simulink library "dlbsBlockTanh"  (R2025b)
settings: Solver=VariableStepAuto  StartTime=0.0  StopTime=10.0  RelTol=1e-3
libraries: dlbsBlockExtractGradientGF x1, dlbsBlockInsertGradientGF x1
settings Model: Creator=lt6037  LastModifiedBy=lt6037

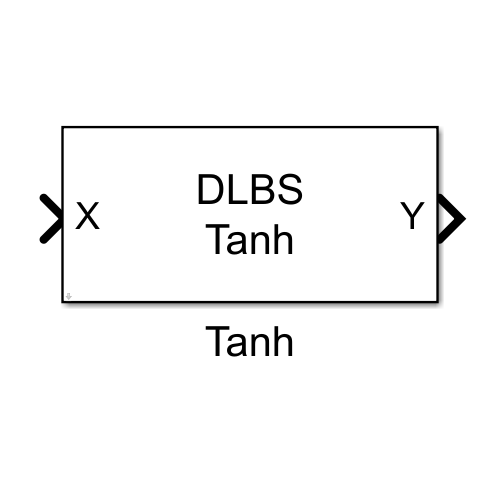
[thumbnail: Simulink's stored preview of the top-level diagram]
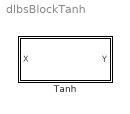
== system dlbsBlockTanh ==
  Tanh : Subsystem
      mask help: Applies the hyperbolic tangent activation to the input tensor. The operation is applied element-wise across all tensor elements.
      mask Help: web("dlbsHelpBlockTanh.html")
      mask Display: fprintf("DLBS\nTanh")

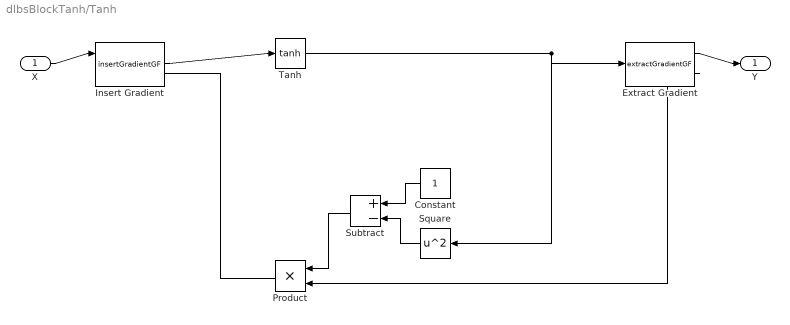
== system dlbsBlockTanh/Tanh ==
  X : Inport
  Constant : Constant
  Extract Gradient : dlbsBlockExtractGradientGF/extractGradientGF
  Insert Gradient : dlbsBlockInsertGradientGF/insertGradientGF
  Product : Product
  Square : Math  Operator=square
  Subtract : Sum  Inputs=+-
  Tanh : Trigonometry  Operator=tanh
  Y : Outport
  wires:
  Constant/1 -> Subtract/1
  Square/1 -> Subtract/2
  Subtract/1 -> Product/1
  Tanh/1 -> Extract Gradient/1, Square/1
  Insert Gradient/1 -> Tanh/1
  Product/1 -> Insert Gradient/2
  Extract Gradient/2 -> Product/2
  X/1 -> Insert Gradient/1
  Extract Gradient/1 -> Y/1
